simulink model "cessna_model"  (R2013a)
settings: Solver=ode45  StartTime=0.0  StopTime=300  RelTol=1e-3
values from neighbouring files (symbols this model uses):
  alpha0 = 0    [cessna_gliding.m]    (also in cessna_powered.m)
  c = 4.9*0.3048    (= 1.49352)    [cessna_gliding.m]    (also in cessna_powered.m)
  CDM = 0.0223    [cessna_gliding.m]    (also in cessna_powered.m)
  CL0 = 0.307    [cessna_gliding.m]    (also in cessna_powered.m)
  CLalpha = 4.41    [cessna_gliding.m]    (also in cessna_powered.m)
  CLalpha_dot = 1.7    [cessna_gliding.m]    (also in cessna_powered.m)
  CLDM = 0    [cessna_gliding.m]    (also in cessna_powered.m)
  CLel = 0.43    [cessna_gliding.m]    (also in cessna_powered.m)
  CLq = 3.9    [cessna_gliding.m]    (also in cessna_powered.m)
  CM0_R = 0.04    [cessna_gliding.m]    (also in cessna_powered.m)
  CMalpha_dot_R = -7.27    [cessna_gliding.m]    (also in cessna_powered.m)
  CMalpha_R = -0.613    [cessna_gliding.m]    (also in cessna_powered.m)
  CMel_R = -1.122    [cessna_gliding.m]    (also in cessna_powered.m)
  CMq_R = -12.4    [cessna_gliding.m]    (also in cessna_powered.m)
  el = 0    [cessna_gliding.m]    (also in cessna_powered.m = 0.0278)
  eT = 0    [cessna_gliding.m]    (also in cessna_powered.m)
  h0 = 1000    [cessna_gliding.m]    (also in cessna_powered.m)
  J2 = 1346*1.35581795    (= 1824.9309607)    [cessna_gliding.m]    (also in cessna_powered.m)
  k = 0.0554    [cessna_gliding.m]    (also in cessna_powered.m)
  m = W/g    (= 1201.60930612)    [cessna_gliding.m]    (also in cessna_powered.m)
  nu = 0.7    [cessna_gliding.m]    (also in cessna_powered.m)
  p0 = 0    [cessna_gliding.m]    (also in cessna_powered.m)
  q0 = 0    [cessna_gliding.m]    (also in cessna_powered.m)
  rho = 1.225    [cessna_gliding.m]    (also in cessna_powered.m)
  S = 174*0.092903    (= 16.165122)    [cessna_gliding.m]    (also in cessna_powered.m)
  th = 0    [cessna_gliding.m]    (also in cessna_powered.m = 74569.9872)
  theta0 = 0    [cessna_gliding.m]    (also in cessna_powered.m)
  V0 = 45    [cessna_gliding.m]    (also in cessna_powered.m)
  W = 2650*4.44822162    (= 11787.787293)    [cessna_gliding.m]    (also in cessna_powered.m)
  xcm = 0    [cessna_gliding.m]    (also in cessna_powered.m)
settings Model: Creator=Willdog  LastModifiedBy=Willdog

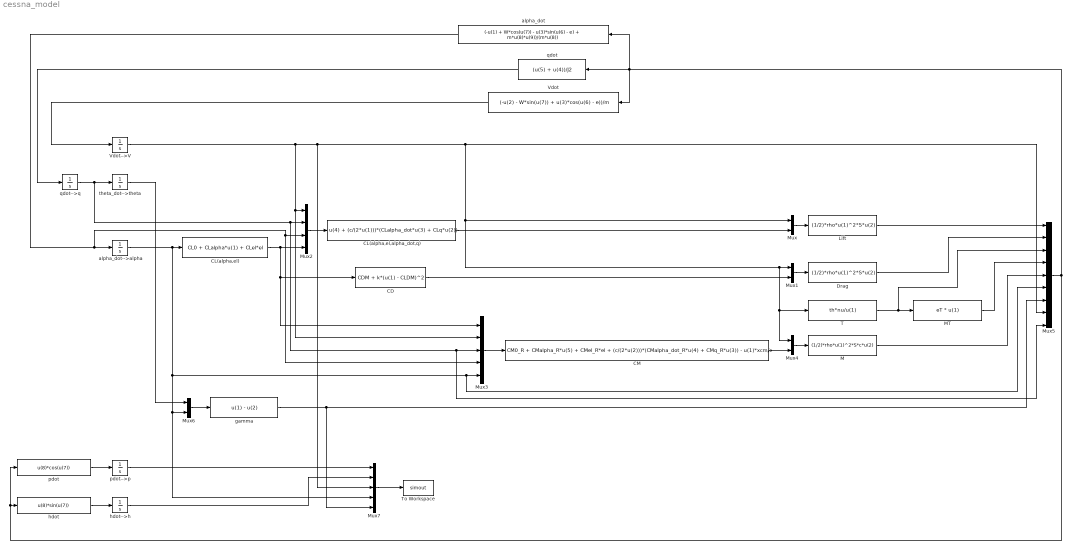
== system cessna_model ==
  CD : Fcn  Expr=CDM + k*(u(1) - CLDM)^2
  CL(alpha,el) : Fcn  Expr=CL0 + CLalpha*u(1) + CLel*el
  CL(alpha,el,alpha_dot,q) : Fcn  Expr=u(4) + (c/(2*u(1)))*(CLalpha_dot*u(3) + CLq*u(2))
  CM : Fcn  Expr=CM0_R + CMalpha_R*u(5) + CMel_R*el + (c/(2*u(2)))*(CMalpha_dot_R*u(4) + CMq_R*u(3)) - u(1)*xcm/c
  Drag : Fcn  Expr=(1/2)*rho*u(1)^2*S*u(2)
  Lift : Fcn  Expr=(1/2)*rho*u(1)^2*S*u(2)
  M : Fcn  Expr=(1/2)*rho*u(1)^2*S*c*u(2)
  MT : Fcn  Expr=eT * u(1)
  Mux{,1,4,6} (4 alike) : Mux  Inputs=2
  Mux2 : Mux
  Mux3 : Mux  Inputs=5
  Mux5 : Mux  Inputs=9
  Mux7 : Mux  Inputs=5
  T : Fcn  Expr=th*nu/u(1)
  To Workspace : ToWorkspace  VariableName=simout  SampleTime=-1  SaveFormat=Timeseries
  Vdot : Fcn  Expr=(-u(2) - W*sin(u(7)) + u(3)*cos(u(6) - e))/m
  Vdot-->V : Integrator  InitialCondition=V0
  alpha_dot : Fcn  Expr=(-u(1) + W*cos(u(7)) - u(3)*sin(u(6) - e) + m*u(8)*u(9))/(m*u(8))
  alpha_dot-->alpha : Integrator  InitialCondition=alpha0
  gamma : Fcn  Expr=u(1) - u(2)
  hdot : Fcn  Expr=u(8)*sin(u(7))
  hdot-->h : Integrator  InitialCondition=h0
  pdot : Fcn  Expr=u(8)*cos(u(7))
  pdot-->p : Integrator  InitialCondition=p0
  qdot : Fcn  Expr=(u(5) + u(4))/J2
  qdot-->q : Integrator  InitialCondition=q0
  theta_dot-->theta : Integrator  InitialCondition=theta0
  wires:
  qdot-->q/1 -> Mux5/9, Mux3/3, Mux2/2, theta_dot-->theta/1
  alpha_dot-->alpha/1 -> Mux7/4, Mux6/2, Mux5/6, Mux3/5, CL(alpha,el)/1
  CL(alpha,el)/1 -> Mux2/4, Mux3/1, CD/1
  Vdot-->V/1 -> Mux7/3, Mux5/8, Mux/1, Mux4/1, T/1, Mux1/1, Mux3/2, Mux2/1
  Mux/1 -> Lift/1
  Mux1/1 -> Drag/1
  CD/1 -> Mux1/2
  Mux2/1 -> CL(alpha,el,alpha_dot,q)/1
  CL(alpha,el,alpha_dot,q)/1 -> Mux/2
  alpha_dot/1 -> Mux3/4, Mux2/3, alpha_dot-->alpha/1
  Mux3/1 -> CM/1
  Mux4/1 -> M/1
  CM/1 -> Mux4/2
  T/1 -> Mux5/3, MT/1
  Lift/1 -> Mux5/1
  Drag/1 -> Mux5/2
  MT/1 -> Mux5/4
  M/1 -> Mux5/5
  Mux5/1 -> alpha_dot/1, Vdot/1, qdot/1, pdot/1, hdot/1
  qdot/1 -> qdot-->q/1
  Vdot/1 -> Vdot-->V/1
  Mux6/1 -> gamma/1
  theta_dot-->theta/1 -> Mux6/1
  gamma/1 -> Mux5/7, Mux7/5
  pdot/1 -> pdot-->p/1
  hdot/1 -> hdot-->h/1
  pdot-->p/1 -> Mux7/1
  hdot-->h/1 -> Mux7/2
  Mux7/1 -> To Workspace/1
